simulink model "compute_speed"  (R2025b)
settings: Solver=FixedStepAuto  StartTime=0.0  StopTime=Tend  FixedStep=Tsim  RelTol=1e-4
values from neighbouring files (symbols this model uses):
  b = 4.28e-6    (= 4.28e-06)    [setup.m]    (also in test.m)
  b_o_sf = wb_sf*J_z    (= 0.00185605293974)    [setup.m]
  J_z = 29.54e-6    (= 2.954e-05)    [setup.m]
  K_io_sf = wb_sf*b    (= 0.000268920331147)    [setup.m]
  Ki_speed = omega_b_speed*b    (= 0.00268920331147)    [setup.m]
  Kp_speed = omega_b_speed*J_z    (= 0.0185605293974)    [setup.m]
  omega_lpf = 2*pi*f_lpf    (= 628.318530718)    [setup.m]
  pole_1_Hz = -10    [computing_speed.m]    (also in setup.m)
  pole_2_Hz = -100    [computing_speed.m]    (also in setup.m)
  speed_cmd = 3000    [setup.m]
  Ts = 1e-4    (= 0.0001)    [setup.m]    (also in test.m = 0.001)
undefined symbols (not defined in the file or in its folder): DiscIntNeverNeededParam
settings Model: Creator=puroh  LastModifiedBy=tnoguchi
settings OptimizationCC: DefaultParameterBehavior=Inlined  EnhancedBackFolding=on  PassReuseOutputArgsAs=Individual arguments  ZeroExternalMemoryAtStartup=off  ZeroInternalMemoryAtStartup=off  OptimizeBlockOrder=speed  DifferentSizesBufferReuse=on  EfficientTunableParamExpr=on
settings DebuggingCC: ParameterTunabilityLossMsg=error  UnconnectedInputMsg=warning  UnconnectedOutputMsg=warning  UnconnectedLineMsg=warning
settings ModelReferenceCC: EnableRefExpFcnMdlSchedulingChecks=on
settings SFSimCC: MATLABDynamicMemAlloc=off
settings RTWCC: SystemTargetFile=ert.tlc  TemplateMakefile=ert_default_tmf  GPUComputeCapability=3.5  DLArmComputeVersion=19.05  Description=Embedded Coder
settings CodeAppCC: ForceParamTrailComments=on  IgnoreCustomStorageClasses=off  OperatorAnnotations=on  SimulinkDataObjDesc=on  SFDataObjDesc=on  InsertBlockDesc=on
settings ERTTargetCC: ERTCustomFileTemplate=example_file_process.tlc  DynamicArrayContainerType=coder::array  TargetLangStandard=C99 (ISO)

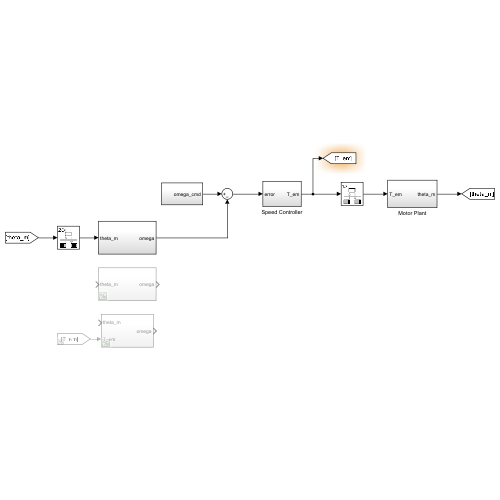
[thumbnail: Simulink's stored preview of the top-level diagram]
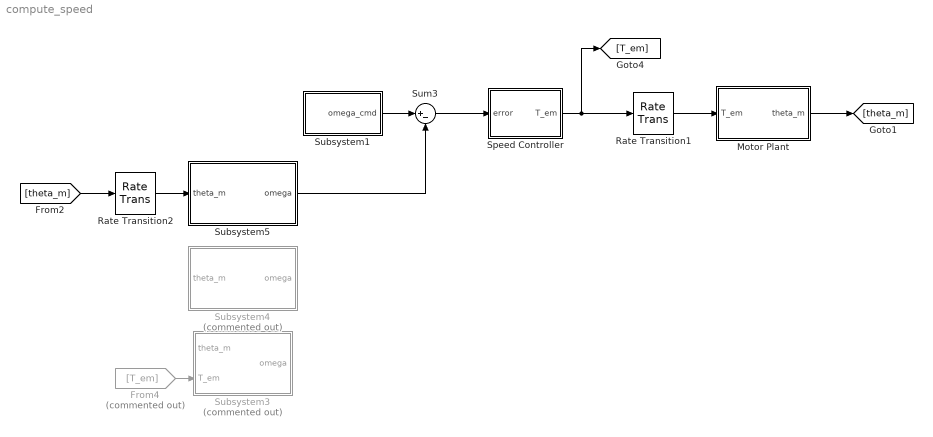
== system compute_speed ==
  From4 : From  Commented=on  GotoTag=T_em
  Motor Plant : Subsystem
  Rate Transition1 : RateTransition
  Rate Transition2 : RateTransition  OutPortSampleTime=Ts
  Speed Controller : Subsystem
  Subsystem1 : Subsystem
  Subsystem3 : Subsystem  Commented=on
  Subsystem4 : Subsystem  Commented=on
  Subsystem5 : Subsystem
  Sum3 : Sum  Inputs=|+-
  wires:
  [theta_m] -> Rate Transition2/1
  Rate Transition1/1 -> Motor Plant/1(T_em)
  Motor Plant/1(theta_m) -> [theta_m]
  Speed Controller/1(T_em) -> Rate Transition1/1, [T_em]
  Subsystem1/1(omega_cmd) -> Sum3/1
  Sum3/1 -> Speed Controller/1(error)
  Rate Transition2/1 -> Subsystem5/1(theta_m)
  Subsystem5/1(omega) -> Sum3/2
  From4/1 -> Subsystem3/2(T_em)

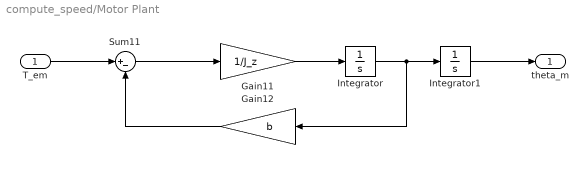
== system compute_speed/Motor Plant ==
  T_em : Inport
  Gain11 : Gain  Gain=1/J_z
  Gain12 : Gain  Gain=b
  Integrator : Integrator
  Integrator1 : Integrator  WrapState=on  WrappedStateUpperValue=2*pi  WrappedStateLowerValue=0
  Sum11 : Sum  Inputs=|+-
  theta_m : Outport
  wires:
  Integrator1/1 -> theta_m/1
  Gain12/1 -> Sum11/2
  Integrator/1 -> Gain12/1, Integrator1/1
  T_em/1 -> Sum11/1
  Gain11/1 -> Integrator/1
  Sum11/1 -> Gain11/1

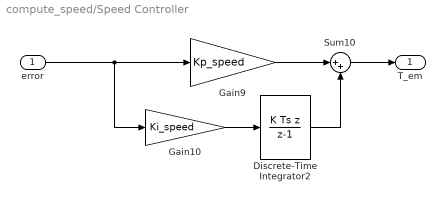
== system compute_speed/Speed Controller ==
  error : Inport
  Discrete-Time Integrator2 : DiscreteIntegrator  IntegratorMethod=Integration: Backward Euler  SampleTime=-1  ICPrevOutput=DiscIntNeverNeededParam  ICPrevScaledInput=DiscIntNeverNeededParam
  Gain10 : Gain  Gain=Ki_speed
  Gain9 : Gain  Gain=Kp_speed
  Sum10 : Sum  Inputs=|++
  T_em : Outport
  wires:
  Discrete-Time Integrator2/1 -> Sum10/2
  Gain9/1 -> Sum10/1
  Gain10/1 -> Discrete-Time Integrator2/1
  error/1 -> Gain10/1, Gain9/1
  Sum10/1 -> T_em/1

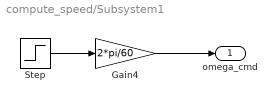
== system compute_speed/Subsystem1 ==
  Gain4 : Gain  Gain=2*pi/60
  Step : Step  Time=0.04  After=speed_cmd  SampleTime=Ts
  omega_cmd : Outport
  wires:
  Step/1 -> Gain4/1
  Gain4/1 -> omega_cmd/1

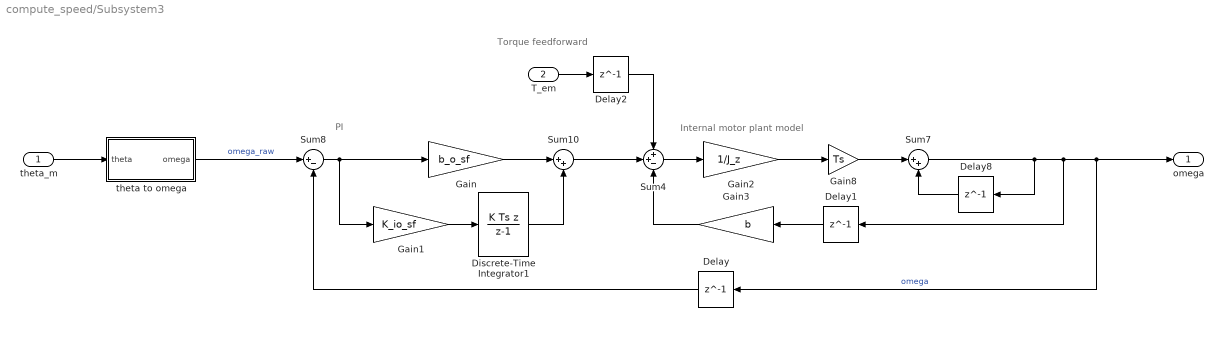
== system compute_speed/Subsystem3 ==
  note: Torque feedforward
  note: PI
  note: Internal motor plant model
  theta_m : Inport
  T_em : Inport  Port=2
  Delay{,1..2,8} (4 alike) : Delay  DelayLength=1  InputProcessing=Columns as channels (frame based)
  Discrete-Time Integrator1 : DiscreteIntegrator  IntegratorMethod=Integration: Backward Euler  SampleTime=-1  ICPrevOutput=DiscIntNeverNeededParam  ICPrevScaledInput=DiscIntNeverNeededParam
  Gain : Gain  Gain=b_o_sf
  Gain1 : Gain  Gain=K_io_sf
  Gain2 : Gain  Gain=1/J_z
  Gain3 : Gain  Gain=b
  Gain8 : Gain  Gain=Ts
  Sum10 : Sum  Inputs=|++
  Sum4 : Sum  Inputs=++-
  Sum7 : Sum  Inputs=|++
  Sum8 : Sum  Inputs=|+-
  theta to omega : Subsystem
  omega : Outport
  wires:
  theta to omega/1(omega) -> Sum8/1  "omega_raw"
  Delay8/1 -> Sum7/2
  Sum8/1 -> Gain1/1, Gain/1
  Gain1/1 -> Discrete-Time Integrator1/1
  Delay/1 -> Sum8/2
  Delay2/1 -> Sum4/1
  Gain/1 -> Sum10/1
  T_em/1 -> Delay2/1
  Sum4/1 -> Gain2/1
  Gain8/1 -> Sum7/1
  Discrete-Time Integrator1/1 -> Sum10/2
  Sum7/1 -> omega/1, Delay/1, Delay1/1, Delay8/1  "omega"
  Sum10/1 -> Sum4/2
  theta_m/1 -> theta to omega/1(theta)
  Gain3/1 -> Sum4/3
  Delay1/1 -> Gain3/1
  Gain2/1 -> Gain8/1

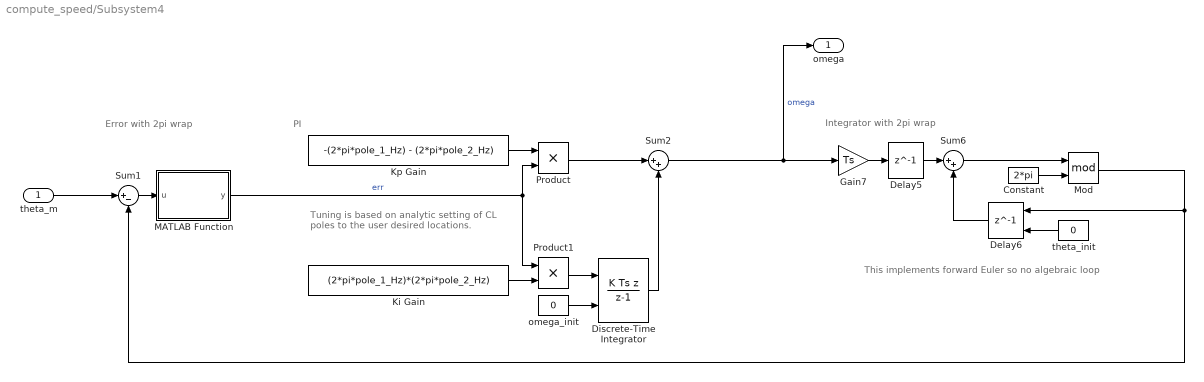
== system compute_speed/Subsystem4 ==
  note: Tuning is based on analytic setting of CL poles to the user desired locations.
  note: PI
  note: Error with 2pi wrap
  note: Integrator with 2pi wrap
  note: This implements forward Euler so no algebraic loop
  theta_m : Inport
  Constant : Constant  Value=2*pi
  Delay5 : Delay  DelayLength=1  InputProcessing=Columns as channels (frame based)
  Delay6 : Delay  DelayLength=1  InitialConditionSource=Input port  InputProcessing=Columns as channels (frame based)
      settings: InputPortMap=u0,p4
  Discrete-Time Integrator : DiscreteIntegrator  IntegratorMethod=Integration: Backward Euler  InitialConditionSource=external  SampleTime=-1  ICPrevOutput=DiscIntNeverNeededParam  ICPrevScaledInput=DiscIntNeverNeededParam
  Gain7 : Gain  Gain=Ts
  Ki Gain : Constant  Value=(2*pi*pole_1_Hz)*(2*pi*pole_2_Hz)
  Kp Gain : Constant  Value=-(2*pi*pole_1_Hz) - (2*pi*pole_2_Hz)
  MATLAB Function : MATLAB Function  TreatAsAtomicUnit=on
  Mod : Math  Operator=mod
  Product : Product
  Product1 : Product
  Sum1 : Sum  Inputs=|+-
  Sum2 : Sum  Inputs=|++
  Sum6 : Sum  Inputs=|++
  omega_init : Constant  Value=0
  theta_init : Constant  Value=0
  omega : Outport
  wires:
  Discrete-Time Integrator/1 -> Sum2/2
  Ki Gain/1 -> Product1/2
  Kp Gain/1 -> Product/1
  Sum6/1 -> Mod/1
  Mod/1 -> Sum1/2, Delay6/1
  Sum1/1 -> MATLAB Function/1(u)
  Delay5/1 -> Sum6/1
  omega_init/1 -> Discrete-Time Integrator/2
  theta_m/1 -> Sum1/1
  Gain7/1 -> Delay5/1
  Delay6/1 -> Sum6/2
  Constant/1 -> Mod/2
  theta_init/1 -> Delay6/2
  Product1/1 -> Discrete-Time Integrator/1
  MATLAB Function/1(y) -> Product1/1, Product/2  "err"
  Product/1 -> Sum2/1
  Sum2/1 -> Gain7/1, omega/1  "omega"

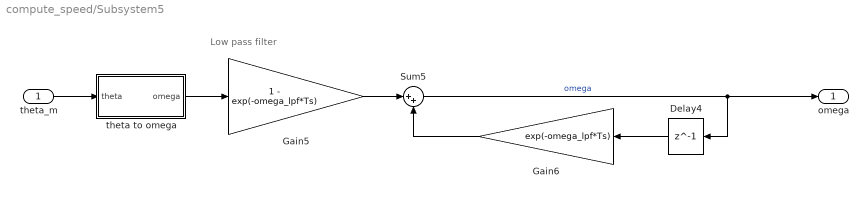
== system compute_speed/Subsystem5 ==
  note: Low pass filter
  theta_m : Inport
  Delay4 : Delay  DelayLength=1  InputProcessing=Columns as channels (frame based)
  Gain5 : Gain  Gain=1 - exp(-omega_lpf*Ts)
  Gain6 : Gain  Gain=exp(-omega_lpf*Ts)
  Sum5 : Sum  Inputs=|++
  theta to omega : Subsystem
  omega : Outport
  wires:
  Delay4/1 -> Gain6/1
  Sum5/1 -> Delay4/1, omega/1  "omega"
  Gain5/1 -> Sum5/1
  Gain6/1 -> Sum5/2
  theta to omega/1(omega) -> Gain5/1
  theta_m/1 -> theta to omega/1(theta)

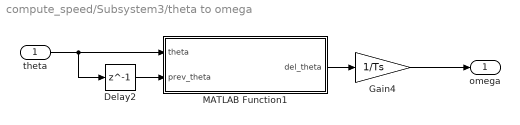
== system compute_speed/Subsystem3/theta to omega ==
  theta : Inport
  Delay2 : Delay  DelayLength=1  InputProcessing=Columns as channels (frame based)
  Gain4 : Gain  Gain=1/Ts
  MATLAB Function1 : MATLAB Function  TreatAsAtomicUnit=on
  omega : Outport
  wires:
  theta/1 -> MATLAB Function1/1(theta), Delay2/1
  Delay2/1 -> MATLAB Function1/2(prev_theta)
  MATLAB Function1/1(del_theta) -> Gain4/1
  Gain4/1 -> omega/1

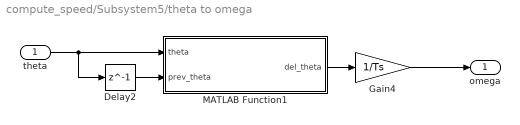
== system compute_speed/Subsystem5/theta to omega ==
  theta : Inport
  Delay2 : Delay  DelayLength=1  InputProcessing=Columns as channels (frame based)
  Gain4 : Gain  Gain=1/Ts
  MATLAB Function1 : MATLAB Function  TreatAsAtomicUnit=on
  omega : Outport
  wires:
  theta/1 -> MATLAB Function1/1(theta), Delay2/1
  Delay2/1 -> MATLAB Function1/2(prev_theta)
  MATLAB Function1/1(del_theta) -> Gain4/1
  Gain4/1 -> omega/1

== matlab function compute_speed/Subsystem5/theta to omega/MATLAB Function1 ==
  data: theta input; del_theta output; prev_theta input
function del_theta = delta_theta(theta, prev_theta)

    % check if prev_theta exist before using to prevent error in 1st iteration 
    del_theta = theta - prev_theta;

    % prevent jumps in speed during 2pi to 0 transitions 
    while del_theta > pi
        del_theta = del_theta - 2*pi;
    end

    while del_theta < -pi
        del_theta = del_theta + 2*pi;
    end
    
end

== matlab function compute_speed/Subsystem4/MATLAB Function ==
  data: u input; y output
function y = fcn(u)

y = u;

if y > pi
    y = y - 2*pi;
end

if y < -pi
    y = y + 2*pi;
end

== matlab function compute_speed/Subsystem3/theta to omega/MATLAB Function1 ==
  data: theta input; del_theta output; prev_theta input
function del_theta = delta_theta(theta, prev_theta)

    % check if prev_theta exist before using to prevent error in 1st iteration 
    del_theta = theta - prev_theta;

    % prevent jumps in speed during 2pi to 0 transitions 
    while del_theta > pi
        del_theta = del_theta - 2*pi;
    end

    while del_theta < -pi
        del_theta = del_theta + 2*pi;
    end
    
end
